simulink model "PMDCmotor"  (R2018a)
settings: Solver=VariableStepAuto  StartTime=0.0  StopTime=0.5  RelTol=1e-3
values from neighbouring files (symbols this model uses):
  Bm = 0.00000604    (= 6.04e-06)    [PMDCparameters.m]    (also in SEDCparameters.m = 1.074e-06; SeriseDCparameters.m = 0.0025; ShuntDCparameters.m = 1.074e-06)
  J = 0.00000161    (= 1.61e-06)    [PMDCparameters.m]    (also in SEDCparameters.m = 0.21; SeriseDCparameters.m = 0.02365; ShuntDCparameters.m = 0.21)
  Kv = 0.0141    [PMDCparameters.m]
  LAA = 0.12    [PMDCparameters.m]    (also in SEDCparameters.m = 0.01; SeriseDCparameters.m; ShuntDCparameters.m = 0.01)
  ra = 7    [PMDCparameters.m]    (also in SEDCparameters.m = 0.013; SeriseDCparameters.m = 1.5; ShuntDCparameters.m = 0.013)
  Tl = 0.003    [PMDCparameters.m]    (also in SEDCparameters.m = 2.493; SeriseDCparameters.m = 10; ShuntDCparameters.m = 2.493)
  Va = 6    [PMDCparameters.m]    (also in SEDCparameters.m = 24; SeriseDCparameters.m = 100; ShuntDCparameters.m = 24)
libraries: fl_lib x11, nesl_utility x6, powerlib x3
settings Model: Creator=Noor  LastModifiedBy=Noor

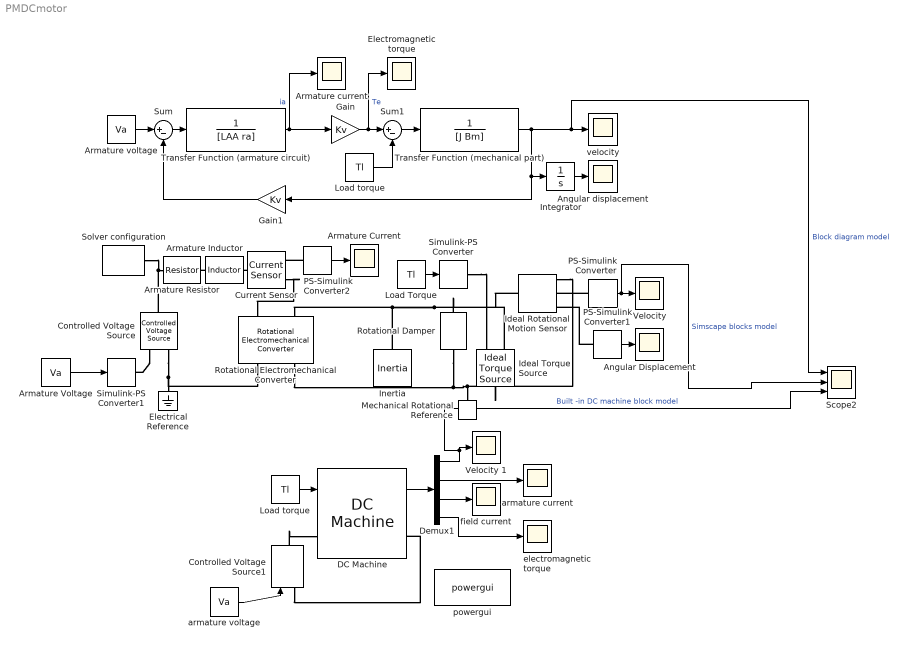
== system PMDCmotor ==
  "    Rotational Electromechanical Converter" : fl_lib/Electrical/Electrical Elements/Rotational Electromechanical Converter  K=Kv V/(rad/s)  i_specify=off  i_priority=None  i=0 A  i_nominal_specify=off  i_nominal_unit=A  i_nominal_value=1  v_specify=off  v_priority=None  v=0 V  v_nominal_specify=off  v_nominal_unit=V  v_nominal_value=1  t_specify=off  t_priority=None  t=0 N*m  t_nominal_specify=off  t_nominal_unit=N*m  t_nominal_value=1  w_specify=off  w_priority=None  w=0 rad/s  w_nominal_specify=off  w_nominal_unit=rad/s  w_nominal_value=1
      settings: SourceProductName=Simscape
  "  Ideal Torque Source" : fl_lib/Mechanical/Mechanical Sources/Ideal Torque Source
  Angular Displacement : Scope
  Angular displacement : Scope
  Armature Voltage : Constant  Value=Va
  Armature current : Scope
  Armature voltage : Constant  Value=Va
  Armature Inductor : fl_lib/Electrical/Electrical Elements/Inductor  l=LAA H  r=0 Ohm  g=0 1/Ohm  i_specify=off  i_priority=None  i=0 A  i_nominal_specify=off  i_nominal_unit=A  i_nominal_value=1  v_specify=off  v_priority=None  v=0 V  v_nominal_specify=off  v_nominal_unit=V  v_nominal_value=1  i_L_specify=off  i_L_priority=High  i_L=0 A  i_L_nominal_specify=off  i_L_nominal_unit=A  i_L_nominal_value=1
  Armature Current : Scope
  Armature Resistor : fl_lib/Electrical/Electrical Elements/Resistor  R=ra Ohm  i_specify=off  i_priority=None  i=0 A  i_nominal_specify=off  i_nominal_unit=A  i_nominal_value=1  v_specify=off  v_priority=None  v=0 V  v_nominal_specify=off  v_nominal_unit=V  v_nominal_value=1
  Controlled Voltage Source : fl_lib/Electrical/Electrical Sources/Controlled Voltage Source
  Controlled Voltage Source1 : powerlib/Electrical Sources/Controlled Voltage Source  Initialize=off  Source_Type=DC  Amplitude=6  Phase=0  Frequency=0  Measurements=None
  Current Sensor : fl_lib/Electrical/Electrical Sensors/Current Sensor
  DC Machine : powerlib/Machines/DC Machine  PresetModel=No  MechanicalLoad=Torque TL  FieldType=Permanent magnet  ShowDetailedParameters=on  MeasurementBus=off  RLa="[ra  LAA]"  RLf="[ 240  120]"  Laf=1.8  MachineConstant=Torque constant (N.m/A)  Ke=Kt  Kt=Kv  J=J  Bm=Bm  Tf=0  w0=0  Ifinit=1  TsPowergui=0  TsBlock=-1
  Demux1 : Demux
  Electrical Reference : fl_lib/Electrical/Electrical Elements/Electrical Reference
  "Electromagnetic torque " : Scope
  Gain : Gain  Gain=Kv
  Gain1 : Gain  Gain=Kv
  Ideal Rotational Motion Sensor : fl_lib/Mechanical/Mechanical Sensors/Ideal Rotational Motion Sensor  offset=0 rad
  "Inertia " : fl_lib/Mechanical/Rotational Elements/Inertia  inertia=J kg*m^2  w_specify=off  w_priority=High  w=0 rad/s  w_nominal_specify=off  w_nominal_unit=rad/s  w_nominal_value=1  t_specify=off  t_priority=None  t=0 N*m  t_nominal_specify=off  t_nominal_unit=N*m  t_nominal_value=1
  Integrator : Integrator
  Load torque : Constant  Value=Tl
  Load Torque : Constant  Value=Tl
  Load torque : Constant  Value=Tl
  Mechanical Rotational Reference : fl_lib/Mechanical/Rotational Elements/Mechanical Rotational Reference
  PS-Simulink Converter : nesl_utility/PS-Simulink Converter  PhysicalDomain=network_engine_domain  SubClassName=ps_output  LeftPortType=input  RightPortType=output  PseudoPeriodic=off  Frequencies=[]  Unit=1  AffineConversion=off
  PS-Simulink Converter1 : nesl_utility/PS-Simulink Converter  PhysicalDomain=network_engine_domain  SubClassName=ps_output  LeftPortType=input  RightPortType=output  PseudoPeriodic=off  Frequencies=[]  Unit=1  AffineConversion=off
  PS-Simulink Converter2 : nesl_utility/PS-Simulink Converter  PhysicalDomain=network_engine_domain  SubClassName=ps_output  LeftPortType=input  RightPortType=output  PseudoPeriodic=off  Frequencies=[]  Unit=1  AffineConversion=off
  Rotational Damper : fl_lib/Mechanical/Rotational Elements/Rotational Damper  D=Bm N*m/(rad/s)  w_specify=off  w_priority=None  w=0 rad/s  w_nominal_specify=off  w_nominal_unit=rad/s  w_nominal_value=1  t_specify=off  t_priority=None  t=0 N*m  t_nominal_specify=off  t_nominal_unit=N*m  t_nominal_value=1
  Scope2 : Scope  NumInputPorts=3
  Simulink-PS Converter : nesl_utility/Simulink-PS Converter  PhysicalDomain=network_engine_domain  SubClassName=ps_input  LeftPortType=input  RightPortType=output  PseudoPeriodic=off  Frequencies=[]  NoiseDistribution=none  NoiseParameters=[]  Unit=1  AffineConversion=off  FilteringAndDerivatives=provide  SimscapeFilterOrder=1  InputFilterTimeConstant=0.001  UdotUserProvided=0
  Simulink-PS Converter1 : nesl_utility/Simulink-PS Converter  PhysicalDomain=network_engine_domain  SubClassName=ps_input  LeftPortType=input  RightPortType=output  PseudoPeriodic=off  Frequencies=[]  NoiseDistribution=none  NoiseParameters=[]  Unit=1  AffineConversion=off  FilteringAndDerivatives=provide  SimscapeFilterOrder=1  InputFilterTimeConstant=0.001  UdotUserProvided=0
  Solver configuration : nesl_utility/Solver Configuration  PhysicalDomain=network_engine_domain  SubClassName=solver  LeftPortType=input  RightPortType=generic  Tones=[]  Harmonics=[]  SimulateNoise=off  Profile=off  UseLocalSampling=off  EnableSwitchedLinearOptims=on  FrequencyDomain=off  UseCCode=off  RelTol=0.001  AbsTol=1e-06  MinStep=1e-09  ToWorkspace=off  RevertToSquareIcSolve=off  NumHomotopyIterations=100  PhasorMode=off  PhasorModeNumHarmonics=1  DoDC=off  ResidualTolerance=1e-09  UseLocalSolver=off  LocalSolverChoice=NE_BACKWARD_EULER_ADVANCER  LocalSolverSampleTime=0.001  DoFixedCost=off  MaxNonlinIter=3  MaxModeIter=2  LinearAlgebra=Sparse  EquationFormulation=NE_TIME_EF  DelaysMemoryBudget=1024  AutomaticFiltering=on  FilteringTimeConstant=0.001
  Sum : Sum  Inputs=|+-
  Sum1 : Sum  Inputs=|+-
  Transfer Function (armature circuit) : TransferFcn  Denominator=[LAA ra]
  Transfer Function (mechanical part) : TransferFcn  Denominator=[J Bm]
  Velocity : Scope
  Velocity 1 : Scope
  armature voltage : Constant  Value=Va
  armature current : Scope
  "electromagnetic torque " : Scope
  field current : Scope
  powergui : powerlib/powergui  Priority=1  SimulationMode=Continuous  SampleTime=50e-6  frequency=60  Iterations=50  frequencyindice=0  Pbase=100e6  ErrMax=1e-4  UnitsV=kV  UnitsW=MW  buscounter=0  FunctionMessages=off  echomessages=off  EnableUseOfTLC=off  CurrentSourceSwitches=off  DisableSnubberDevices=off  DisableRonSwitches=off  DisableVfSwitches=off  DisplayEquations=off  SolverType=Tustin/Backward Euler (TBE)  Interpol=off  ExternalGateDelay=off  methode=off  Ts=100  x0status=blocks  SPID=on  SwTol=0  HookPort=off  RestoreLinks=warning  ResistiveCurrentMeasurement=off  Frange=[0:2:500]  Ylog=off  Xlog=on  ShowGrid=off  save=off  variable=ZData  structure=0  ZoomFFT=off  StartTime=0.0  cycles=1  DisplayStyle=1  fundamental=60  FreqAxis=off  MaxFrequency=1000  frequencyindicesteady=1  RmsSteady=1  display=off
  velocity : Scope
  wires:
  Gain/1 -> Sum1/1, "Electromagnetic torque "/1  "Te"
  Transfer Function (armature circuit)/1 -> Gain/1, Armature current/1  "ia"
  Sum/1 -> Transfer Function (armature circuit)/1
  Sum1/1 -> Transfer Function (mechanical part)/1
  Transfer Function (mechanical part)/1 -> Scope2/1, velocity/1, Integrator/1, Gain1/1  "Block diagram model"
  Gain1/1 -> Sum/2
  Armature voltage/1 -> Sum/1
  Integrator/1 -> Angular displacement/1
  Load torque/1 -> Sum1/2
  PS-Simulink Converter2/1 -> Armature Current/1
  Load Torque/1 -> Simulink-PS Converter/1
  PS-Simulink Converter1/1 -> Angular Displacement/1
  PS-Simulink Converter/1 -> Scope2/2, Velocity/1  "Simscape blocks model"
  Demux1/3 -> field current/1
  Demux1/1 -> Scope2/3, Velocity 1/1  "Built -in DC machine block model"
  Demux1/4 -> "electromagnetic torque "/1
  DC Machine/1 -> Demux1/1
  Demux1/2 -> armature current/1
  Load torque/1 -> DC Machine/1
  Armature Voltage/1 -> Simulink-PS Converter1/1
  armature voltage/1 -> Controlled Voltage Source1/1
  connections:
  Armature Inductor/LConn1 -- Armature Resistor/RConn1
  "Inertia "/LConn1 -- Rotational Damper/LConn1 -- Ideal Rotational Motion Sensor/LConn1 -- "  Ideal Torque Source"/RConn2 -- "    Rotational Electromechanical Converter"/LConn2
  "    Rotational Electromechanical Converter"/RConn2 -- Rotational Damper/RConn1 -- Ideal Rotational Motion Sensor/RConn1 -- "  Ideal Torque Source"/LConn1 -- Mechanical Rotational Reference/LConn1
  Simulink-PS Converter/RConn1 -- "  Ideal Torque Source"/RConn1
  Controlled Voltage Source/LConn1 -- Armature Resistor/LConn1 -- Solver configuration/RConn1
  Controlled Voltage Source/RConn2 -- "    Rotational Electromechanical Converter"/RConn1 -- Electrical Reference/LConn1
  PS-Simulink Converter/LConn1 -- Ideal Rotational Motion Sensor/RConn2
  PS-Simulink Converter1/LConn1 -- Ideal Rotational Motion Sensor/RConn3
  Current Sensor/LConn1 -- Armature Inductor/RConn1
  Current Sensor/RConn2 -- "    Rotational Electromechanical Converter"/LConn1
  PS-Simulink Converter2/LConn1 -- Current Sensor/RConn1
  Controlled Voltage Source/RConn1 -- Simulink-PS Converter1/RConn1
  Controlled Voltage Source1/RConn1 -- DC Machine/LConn1
  Controlled Voltage Source1/LConn1 -- DC Machine/RConn1
